simulink model "mg615503"  (Simulink 7.6)
settings: Solver=FixedStepDiscrete  StartTime=0.0  StopTime=10.0  RelTol=1e-3
PreLoadFcn:
  | REG = mpt.Signal;
  | REG.DataType = 'single';
  | REG.Dimensions = 4;
libraries: simulink x4
settings Model: Creator=kgrand  LastModifiedBy=pnichols
settings OptimizationCC: InlineParams=on  UseIntDivNetSlope=on  InlineInvariantSignals=on  EnhancedBackFolding=on  EfficientFloat2IntCast=on  OptimizeModelRefInitCode=on  LifeSpan=1  AccelVerboseBuild=on
settings RTWCC: SystemTargetFile=ert.tlc  GenCodeOnly=on  TemplateMakefile=ert_default_tmf  Description=Real-Time Workshop Embedded Coder  ProcessScript=ert_make_rtw_hook
settings CodeAppCC: IgnoreCustomStorageClasses=off
settings ERTTargetCC: MultiwordLength=2048  GenerateSampleERTMain=on  GenerateSLWebview=off  InlinedParameterPlacement=NonHierarchical  ERTCustomFileTemplate=example_file_process.tlc  ConvertIfToSwitch=off

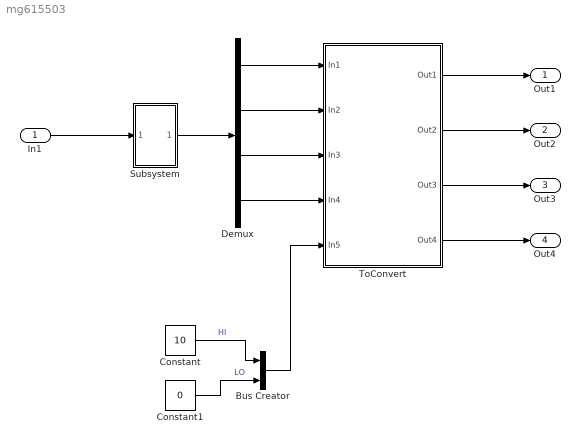
== system mg615503 ==
  In1 : Inport
  Bus Creator : BusCreator  Inputs=2
  Constant : Constant  Value=10  OutDataTypeStr=single  SampleTime=-1
  Constant1 : Constant  Value=0  OutDataTypeStr=single  SampleTime=-1
  Demux : Demux
  Subsystem : Subsystem  TreatAsAtomicUnit=on
  ToConvert : Subsystem  TreatAsAtomicUnit=on
  Out1 : Outport
  Out2 : Outport  Port=2
  Out3 : Outport  Port=3
  Out4 : Outport  Port=4
  wires:
  In1/1 -> Subsystem/1(In1)
  ToConvert/1(Out1) -> Out1/1
  Demux/1 -> ToConvert/1(In1)
  Subsystem/1(Out1) -> Demux/1
  Constant/1 -> Bus Creator/1  "HI"
  Constant1/1 -> Bus Creator/2  "LO"
  Bus Creator/1 -> ToConvert/5(In5)
  Demux/2 -> ToConvert/2(In2)
  Demux/3 -> ToConvert/3(In3)
  Demux/4 -> ToConvert/4(In4)
  ToConvert/2(Out2) -> Out2/1
  ToConvert/3(Out3) -> Out3/1
  ToConvert/4(Out4) -> Out4/1

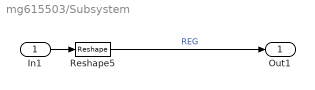
== system mg615503/Subsystem ==
  In1 : Inport
  Reshape5 : Reshape
  Out1 : Outport
  wires:
  In1/1 -> Reshape5/1
  Reshape5/1 -> Out1/1  "REG"

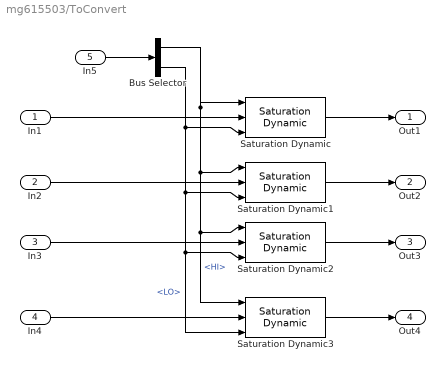
== system mg615503/ToConvert ==
  In1 : Inport
  In2 : Inport  Port=2
  In3 : Inport  Port=3
  In4 : Inport  Port=4
  In5 : Inport  Port=5
  Bus Selector : BusSelector  OutputSignals=HI,LO
  Saturation Dynamic{,1..3} (4 alike) : simulink/Discontinuities/Saturation Dynamic  SystemSampleTime=-1  OutMin=[]  OutMax=[]  OutDataTypeStr=Inherit: Same as second input  OutDataType=fixdt(1, 16)  OutScaling=2^-10  DoSatur=off
  Out1 : Outport
  Out2 : Outport  Port=2
  Out3 : Outport  Port=3
  Out4 : Outport  Port=4
  wires:
  In1/1 -> Saturation Dynamic/2
  Saturation Dynamic/1 -> Out1/1
  In5/1 -> Bus Selector/1
  Bus Selector/1 -> Saturation Dynamic3/1, Saturation Dynamic2/1, Saturation Dynamic1/1, Saturation Dynamic/1  "<HI>"
  Bus Selector/2 -> Saturation Dynamic3/3, Saturation Dynamic2/3, Saturation Dynamic1/3, Saturation Dynamic/3  "<LO>"
  In2/1 -> Saturation Dynamic1/2
  Saturation Dynamic1/1 -> Out2/1
  Saturation Dynamic2/1 -> Out3/1
  In4/1 -> Saturation Dynamic3/2
  Saturation Dynamic3/1 -> Out4/1
  In3/1 -> Saturation Dynamic2/2
